simulink model "simple_router_3D"  (R2015a)
settings: Solver=ode45  StartTime=0.0  StopTime=10.0  RelTol=1e-3
undefined symbols (not defined in the file or in its folder): des
settings Model: Creator=Nejib  LastModifiedBy=Nejib

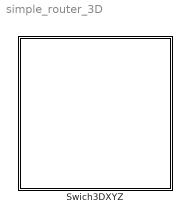
== system simple_router_3D ==
  Swich3DXYZ : Subsystem  mask{ME_X=1, ME_Y=1, ME_Z=1, C=16, D=1, F=1, S=1e-6}
      mask prompts: ME_X "X"; ME_Y "Y"; ME_Z "Z"; C "Input FIFO size in flits"; D "Routing and arbitration delay"; F "Clock Frequency"; S "Standard Deviation"
      mask DialogControl DescTextVar Prompt: 7 Port router with the XYZ routing algorithm.
      mask DialogControl Container6 Prompt: Address

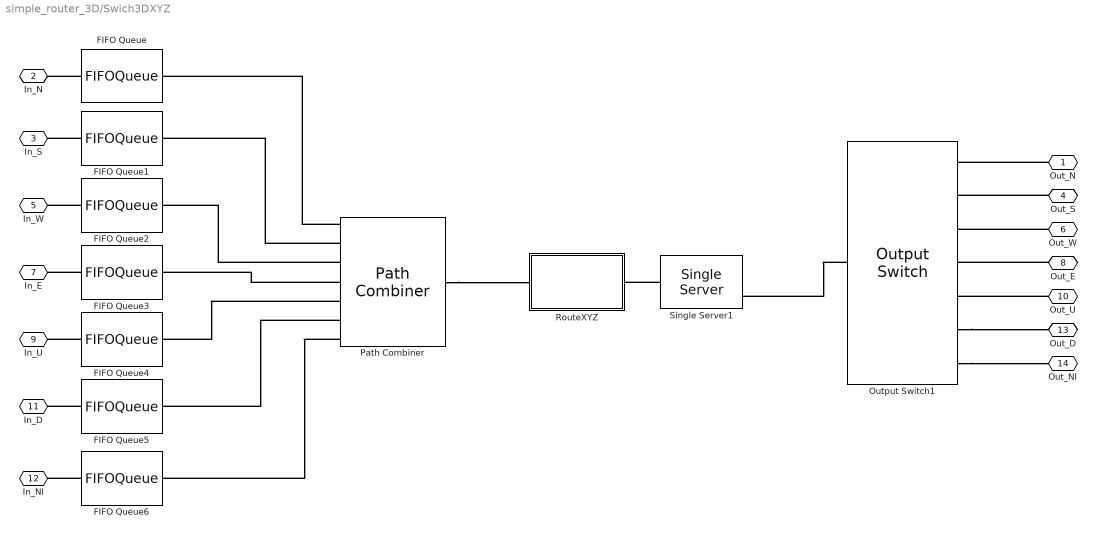
== system simple_router_3D/Swich3DXYZ ==
  FIFO Queue{,1..6} (7 alike) : FIFOQueue
  Output Switch1 : OutputSwitch  NumberOutputPorts=7  SwitchingCriterion=From attribute  AttributeName=RT  InitialConditionsOpt=on  InitialConditions=5
  Path Combiner : PathCombiner  NumberInputPorts=7  InputPortPrecedence=Equiprobable  InitialSeed=4648
  RouteXYZ : Subsystem
  Single Server1 : SingleServer  ServiceTime=D  StatNumberDeparted=on
  Out_N : PMIOPort  Port=1  Side=Right
  In_N : PMIOPort  Port=2  Side=Left
  In_S : PMIOPort  Port=3  Side=Left
  Out_S : PMIOPort  Port=4  Side=Right
  In_W : PMIOPort  Port=5  Side=Left
  Out_W : PMIOPort  Port=6  Side=Right
  In_E : PMIOPort  Port=7  Side=Left
  Out_E : PMIOPort  Port=8  Side=Right
  In_U : PMIOPort  Port=9  Side=Left
  Out_U : PMIOPort  Port=10  Side=Right
  In_D : PMIOPort  Port=11  Side=Left
  In_NI : PMIOPort  Port=12  Side=Left
  Out_D : PMIOPort  Port=13  Side=Right
  Out_NI : PMIOPort  Port=14  Side=Right
  connections:
  Single Server1/LConn1 -- RouteXYZ/RConn1
  Path Combiner/RConn1 -- RouteXYZ/LConn1
  FIFO Queue6/LConn1 -- In_NI/RConn1
  FIFO Queue5/LConn1 -- In_D/RConn1
  Output Switch1/RConn7 -- Out_NI/RConn1
  Output Switch1/RConn6 -- Out_D/RConn1
  Path Combiner/LConn7 -- FIFO Queue6/RConn1
  Path Combiner/LConn6 -- FIFO Queue5/RConn1
  Out_U/RConn1 -- Output Switch1/RConn5
  Out_E/RConn1 -- Output Switch1/RConn4
  Out_W/RConn1 -- Output Switch1/RConn3
  Out_S/RConn1 -- Output Switch1/RConn2
  Out_N/RConn1 -- Output Switch1/RConn1
  Path Combiner/LConn5 -- FIFO Queue4/RConn1
  Path Combiner/LConn4 -- FIFO Queue3/RConn1
  Path Combiner/LConn3 -- FIFO Queue2/RConn1
  Path Combiner/LConn2 -- FIFO Queue1/RConn1
  Path Combiner/LConn1 -- FIFO Queue/RConn1
  Output Switch1/LConn1 -- Single Server1/RConn1
  FIFO Queue4/LConn1 -- In_U/RConn1
  FIFO Queue/LConn1 -- In_N/RConn1
  FIFO Queue3/LConn1 -- In_E/RConn1
  FIFO Queue2/LConn1 -- In_W/RConn1
  FIFO Queue1/LConn1 -- In_S/RConn1

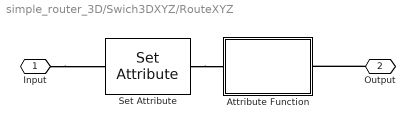
== system simple_router_3D/Swich3DXYZ/RouteXYZ ==
  Attribute Function : Subsystem  LoadFcn=des.afb.attributefunction_support(gcb,'LoadFcn');  StartFcn=des.afb.attributefunction_support(gcb,'StartFcn');  mask(Attribute Function){OutputNamePrefix=out_}
      mask prompts: OutputNamePrefix "Prefix name"
      settings: CopyFcn=des.afb.attributefunction_support(gcb,'CopyFcn');  OpenFcn=des.afb.attributefunction_support(gcb,'OpenFcn');  ErrorFcn=des.afb.error_redirect
      mask Help: slhelp(gcbh)
      mask Display: image(des_iconLoad('attribFunction.jpg'),'center');
  Set Attribute : SetAttribute  AttributeName=IME_X|IME_Y|IME_Z  AttributeFrom=Dialog|Dialog|Dialog  AttributeValue=ME_X|ME_Y|ME_Z  AttributeTreatAsVector=1|1|1  EvaluatedAttributeValue={ ME_X;ME_Y;ME_Z}
  Input : PMIOPort  Port=1  Side=Left
  Output : PMIOPort  Port=2  Side=Right
  connections:
  Input/RConn1 -- Set Attribute/LConn1
  Output/RConn1 -- Attribute Function/RConn1
  Set Attribute/RConn1 -- Attribute Function/LConn1

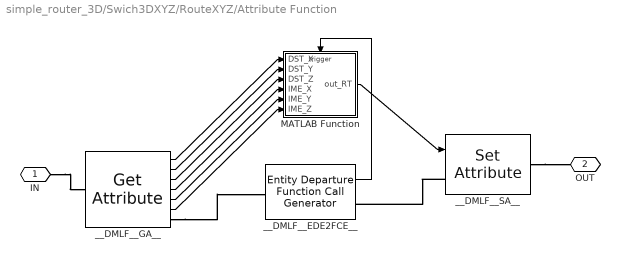
== system simple_router_3D/Swich3DXYZ/RouteXYZ/Attribute Function ==
  MATLAB Function : MATLAB Function  TreatAsAtomicUnit=on
  __DMLF__EDE2FCE__ : EntityDepartureFunctionCallGenerator  TimingFunctionCallF1=Before entity departure  IsInsideAFB=on
  __DMLF__GA__ : GetAttribute  AttributeName=DST_X|DST_Y|DST_Z|IME_X|IME_Y|IME_Z  AttributeMissing=Error|Error|Error|Error|Error|Error  AttributeDefaultValue=1|1|1|1|1|1  AttributeTreatAsVector=1|1|1|1|1|1  AttributeSendTiming=Before entity departure|Before entity departure|Before entity departure|Before entity departure|Before entity departure|Before entity departure  EvaluatedDefaultAttributeValue={ [];[];[];[];[];[]}  IsInsideAFB=on
      settings: OutputPortMap=o1,o2,o3,o4,o5,o6
  __DMLF__SA__ : SetAttribute  AttributeName=RT  AttributeFrom=Signal port  EvaluatedAttributeValue={ []}  IsInsideAFB=on
  IN : PMIOPort  Port=1  Side=Left
  OUT : PMIOPort  Port=2  Side=Right
  wires:
  __DMLF__EDE2FCE__/1 -> MATLAB Function/Trigger
  __DMLF__GA__/1 -> MATLAB Function/1(DST_X)
  __DMLF__GA__/2 -> MATLAB Function/2(DST_Y)
  __DMLF__GA__/3 -> MATLAB Function/3(DST_Z)
  __DMLF__GA__/4 -> MATLAB Function/4(IME_X)
  __DMLF__GA__/5 -> MATLAB Function/5(IME_Y)
  __DMLF__GA__/6 -> MATLAB Function/6(IME_Z)
  MATLAB Function/1(out_RT) -> __DMLF__SA__/1
  connections:
  __DMLF__SA__/RConn1 -- OUT/RConn1
  IN/RConn1 -- __DMLF__GA__/LConn1
  __DMLF__GA__/RConn1 -- __DMLF__EDE2FCE__/LConn1
  __DMLF__SA__/LConn1 -- __DMLF__EDE2FCE__/RConn1

== matlab function simple_router_3D/Swich3DXYZ/RouteXYZ/Attribute Function/MATLAB Function ==
  data: DST_X input; out_RT output; DST_Y input; DST_Z input; IME_X input; IME_Y input; IME_Z input
  events: trigger input FUNCTION_CALL_EVENT
function out_RT  = fcn(DST_X,DST_Y,DST_Z, IME_X, IME_Y,IME_Z)
%FCN    Access and modify attributes with MATLAB 
% 
% Input arguments must match the attribute names.
% Output arguments must be out_<AttributeName>,
% e.g., out_ServiceTime where ServiceTime is the attribute name.
% 
% The output attribute will be created if it is not present.
%

North = 1;
South = 2;
West = 3;
East = 4;
Up = 5;
Down = 6;
NI = 7;

xi =IME_X;
yi =IME_Y;
zi =IME_Z;


x = DST_X;
y = DST_Y;
z = DST_Z;

if (xi ~= x),
    if (xi < x),
        out_RT = West;
    else
        out_RT = East;
    end
elseif (yi ~= y),
    if (yi < y),
        out_RT = North;
    else
        out_RT = South;
    end
elseif (zi ~= z),
    if (zi < z),
        out_RT = Up;
    else
        out_RT = Down;
    end
else
    out_RT = NI;
end
